simulink model "Integrate_SubMode_Motor"  (R2021b)
settings: Solver=FixedStepAuto  StartTime=0.0  StopTime=inf  FixedStep=0.01  RelTol=1e-3  EnableMultiTasking=on
values from neighbouring files (symbols this model uses):
  den_Gd = Gd.Den{:}    [para.m]
  Ki = 0.003    [para.m]
  Kp = 0.0001    [para.m]
  num_Gd = Gd.Num{:}    [para.m]
  rpm_scale = 1/12/4*60    (= 1.25)    [para.m]
  Wref = 4000    [para.m]
undefined symbols (not defined in the file or in its folder): dir, dist, pot2rpm
libraries: arduinolib x8, arduinosensorlib x5, simulink x4
settings Model: SimulationMode=external  ExtModeTrigDuration=2  Creator=user  LastModifiedBy=user
settings SolverCC: AutoInsertRateTranBlk=on
settings OptimizationCC: EnhancedBackFolding=on  PassReuseOutputArgsAs=Individual arguments  ZeroExternalMemoryAtStartup=off  ZeroInternalMemoryAtStartup=off  MaxStackSize=64  OptimizeBlockOrder=speed  DifferentSizesBufferReuse=on  OptimizationCustomize=off  EfficientTunableParamExpr=on
settings DebuggingCC: ParameterTunabilityLossMsg=error
settings HardwareCC: ProdBitPerInt=16  ProdBitPerPointer=16  ProdBitPerSizeT=16  ProdBitPerPtrDiffT=16  ProdLargestAtomicFloat=None  ProdWordSize=8  ProdHWDeviceType=Atmel->AVR
settings SFSimCC: MATLABDynamicMemAlloc=off
settings RTWCC: Description=Embedded Coder  SystemTargetFile=ert.tlc  HardwareBoard=Arduino Mega 2560  TemplateMakefile=ert_default_tmf  Toolchain=Arduino AVR  BuildConfiguration=Faster Runs
settings CodeAppCC: ForceParamTrailComments=on  IgnoreCustomStorageClasses=off  OperatorAnnotations=on  SimulinkDataObjDesc=on  SFDataObjDesc=on  InsertBlockDesc=on
settings ERTTargetCC: SupportContinuousTime=on  SupportVariableSizeSignals=on  ExtMode=on  ExtModeTransport=3  ExtModeStaticAlloc=on  ExtModeStaticAllocSize=2048  ExtModeMexFile=ext_xcp  ExtModeMexArgs=0 5 921600  ExtModeIntrfLevel=Level2 - Open

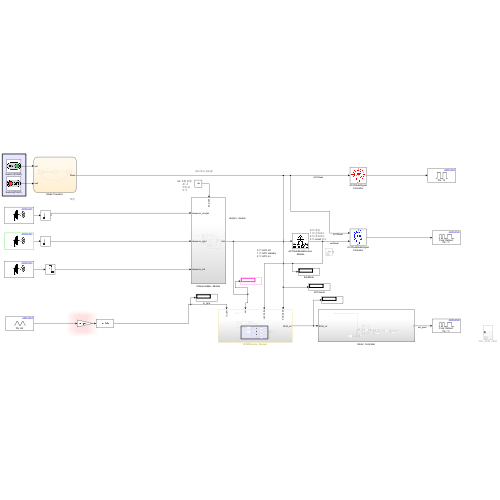
[thumbnail: Simulink's stored preview of the top-level diagram]
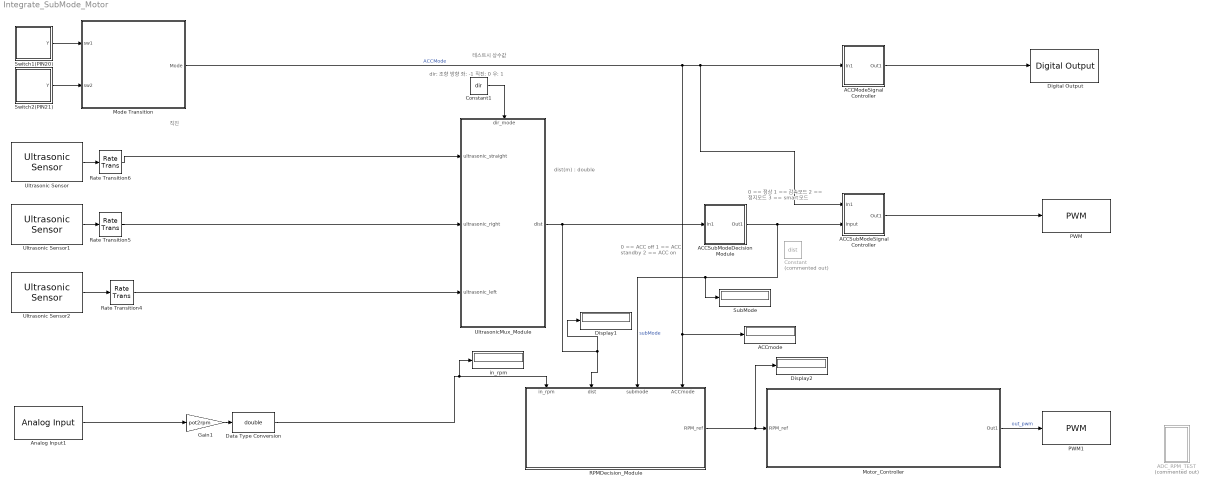
== system Integrate_SubMode_Motor ==
  note: dist(m) : double
  note: 테스트시 상수값
  note: 직진
  note: dir: 조향 방향
      |  	좌: -1
      |  	직진: 0
      |  	우: 1
  note: 0 == 정상
      | 1 == 감속모드
      | 2 == 정지모드
      | 3 == smart 모드
  note: 0 == ACC off
      | 1 == ACC standby
      | 2 == ACC on
  ACCModeSignal Controller : Subsystem
      mask Display: image('$imagefile'); % 변경하려면 툴스트립에 있는 "이미지 편집"을 사용하십시오.
  ACCSubModeDecision Module : Subsystem
      mask Display: image('$imagefile'); % 변경하려면 툴스트립에 있는 "이미지 편집"을 사용하십시오.
  ACCSubModeSignal Controller : Subsystem
      mask Display: image('$imagefile'); % 변경하려면 툴스트립에 있는 "이미지 편집"을 사용하십시오.
  ACCmode : Display
  ADC_RPM_TEST : Subsystem  Commented=on
  Analog Input1 : arduinolib/Analog Input  pinNumber=0  ReadResultsOnly=off  ConversionTriggerSource=Software  ExternalTriggerType=uint32( 0 )  OutputDataType=uint16  EnableConversionCompleteNotify=off  EnableOuputStatus=off  SampleTime=-1  blockPlatform=arduino
  Constant : Constant  Commented=on  Value=dist
  Constant1 : Constant  Value=dir
  Data Type Conversion : DataTypeConversion  OutDataTypeStr=double
  Digital Output : arduinolib/Digital Output  pinNumber=12  Direction=output  blockPlatform=arduino
  Display1 : Display
  Display2 : Display
  Gain1 : Gain  Gain=pot2rpm
  Mode Transition : Stateflow chart  TreatAsAtomicUnit=on
  Motor_Controller : Subsystem
  PWM : arduinolib/PWM  pinNumber=11  frequencyType=Default  desiredFrequency=490.2  achievableFrequency=490.2
  PWM1 : arduinolib/PWM  pinNumber=11  frequencyType=Default  desiredFrequency=490.2  achievableFrequency=490.2
  RPMDecision_Module : Subsystem
      settings: PortSchema="{\"entries\":[{\"content\":{\"sides\":[{\"content\":{\"connectorIds\":[]},\"type\":\"ConnectorPlacement.EquallySpacedRectSide\",\"uuid\":\"6ec364ce-34b2-4beb-b97a-f32003c79d6e\"},{\"content\":{\"connectorIds\":[\"Out1\"],\"side\":\"RIGHT\"},\"type\":\"ConnectorPlacement.EquallySpacedRectSide\",\"uuid\":\"dc876503-cb4c-4ae1-9014-14ad87bdb333\"},{\"content\":{\"connectorIds\":[\"In1\",\"In2\",\"In3\",\"In4\"],\"side\":\"TOP\"},\"type\":\"ConnectorPlacement.EquallySpacedRectSide\",\"uuid\":\"5447802f-a25d-4c34-9dc6-d7b36056ed0d\"}]},\"type\":\"ConnectorPlacement.EquallySpacedConnector\",\"uuid\":\"292fcb4a-6f45-4a66-adbd-fd22b6096994\"}],\"packageUris\":[\"http://schema.mathworks.com/mf0/Connector/R2020b\"],\"version\":\"1.0\"}"
  Rate Transition4 : RateTransition  Deterministic=off  OutPortSampleTime=0.03
  Rate Transition5 : RateTransition  Deterministic=off  OutPortSampleTime=0.03
  Rate Transition6 : RateTransition  Deterministic=off  OutPortSampleTime=0.03
  SubMode : Display
  Switch1(PIN20) : Subsystem
      mask Display: image('$imagefile'); % 변경하려면 툴스트립에 있는 "이미지 편집"을 사용하십시오.
  Switch2(PIN21) : Subsystem
      mask Display: image('$imagefile'); % 변경하려면 툴스트립에 있는 "이미지 편집"을 사용하십시오.
  Ultrasonic Sensor : arduinosensorlib/Ultrasonic Sensor  NumSignalPins=2  TrigPin=50  EchoPin=51  SignalPin=3  SampleTime_=0.1  blockPlatform=ARDUINO
      settings: SourceProductBaseCode=ARDUINO
  Ultrasonic Sensor1 : arduinosensorlib/Ultrasonic Sensor  NumSignalPins=2  TrigPin=48  EchoPin=49  SignalPin=3  SampleTime_=0.1  blockPlatform=ARDUINO
      settings: SourceProductBaseCode=ARDUINO
  Ultrasonic Sensor2 : arduinosensorlib/Ultrasonic Sensor  NumSignalPins=2  TrigPin=46  EchoPin=47  SignalPin=3  SampleTime_=0.1  blockPlatform=ARDUINO
      settings: SourceProductBaseCode=ARDUINO
  UltrasonicMux_Module : Subsystem
      settings: PortSchema="{\"entries\":[{\"content\":{\"sides\":[{\"content\":{\"connectorIds\":[\"In1\",\"In2\",\"In3\"]},\"type\":\"ConnectorPlacement.EquallySpacedRectSide\",\"uuid\":\"5f4ad8f0-04c3-4479-9dfd-33641402f242\"},{\"content\":{\"connectorIds\":[\"Out1\"],\"side\":\"RIGHT\"},\"type\":\"ConnectorPlacement.EquallySpacedRectSide\",\"uuid\":\"c4451af6-64c8-402e-8ffe-feeed5b209e6\"},{\"content\":{\"connectorIds\":[\"In4\"],\"side\":\"TOP\"},\"type\":\"ConnectorPlacement.EquallySpacedRectSide\",\"uuid\":\"4be8f8c7-8102-4379-8072-e8a8027f489d\"}]},\"type\":\"ConnectorPlacement.EquallySpacedConnector\",\"uuid\":\"2bd08bb9-e7f4-4004-b808-4b0f9daf5a96\"}],\"packageUris\":[\"http://schema.mathworks.com/mf0/Connector/R2020b\"],\"version\":\"1.0\"}"
  in_rpm : Display
  wires:
  Gain1/1 -> Data Type Conversion/1
  Data Type Conversion/1 -> in_rpm/1, RPMDecision_Module/1(in_rpm)
  Constant1/1 -> UltrasonicMux_Module/4(dir_mode)
  Ultrasonic Sensor2/1 -> Rate Transition4/1
  Ultrasonic Sensor1/1 -> Rate Transition5/1
  Ultrasonic Sensor/1 -> Rate Transition6/1
  Rate Transition6/1 -> UltrasonicMux_Module/1(ultrasonic_straight)
  Rate Transition5/1 -> UltrasonicMux_Module/2(ultrasonic_right)
  Rate Transition4/1 -> UltrasonicMux_Module/3(ultrasonic_left)
  Analog Input1/1 -> Gain1/1
  Motor_Controller/1(Out1) -> PWM1/1  "out_pwm"
  RPMDecision_Module/1(RPM_ref) -> Display2/1, Motor_Controller/1(RPM_ref)
  UltrasonicMux_Module/1(dist) -> ACCSubModeDecision Module/1(In1), RPMDecision_Module/2(dist), Display1/1
  Switch2(PIN21)/1(Y) -> Mode Transition/2(sw2)
  Switch1(PIN20)/1(Y) -> Mode Transition/1(sw1)
  Mode Transition/1(Mode) -> ACCSubModeSignal Controller/1(In1), ACCModeSignal Controller/1(In1), ACCmode/1, RPMDecision_Module/4(ACCmode)  "ACCMode"
  ACCSubModeDecision Module/1(Out1) -> ACCSubModeSignal Controller/2(Input), RPMDecision_Module/3(submode), SubMode/1  "subMode"
  ACCModeSignal Controller/1(Out1) -> Digital Output/1
  ACCSubModeSignal Controller/1(Out1) -> PWM/1

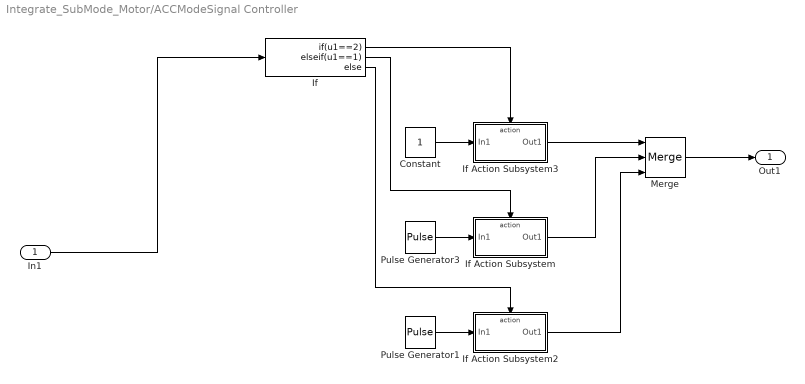
== system Integrate_SubMode_Motor/ACCModeSignal Controller ==
  In1 : Inport
  Constant : Constant
  If : If  IfExpression=u1==2  ElseIfExpressions=u1==1
  If Action Subsystem : Subsystem  TreatAsAtomicUnit=on
  If Action Subsystem2 : Subsystem  TreatAsAtomicUnit=on
  If Action Subsystem3 : Subsystem  TreatAsAtomicUnit=on
  Merge : Merge  Inputs=3
  Pulse Generator1 : DiscretePulseGenerator  PulseType=Time based  Period=1  PulseWidth=50  SampleTime=-1
  Pulse Generator3 : DiscretePulseGenerator  PulseType=Time based  Period=0.2  PulseWidth=50  SampleTime=-1
  Out1 : Outport
  wires:
  If Action Subsystem2/1(Out1) -> Merge/3
  Pulse Generator1/1 -> If Action Subsystem2/1(In1)
  Pulse Generator3/1 -> If Action Subsystem/1(In1)
  Merge/1 -> Out1/1
  If Action Subsystem/1(Out1) -> Merge/2
  If/1 -> If Action Subsystem3/Action
  If/2 -> If Action Subsystem/Action
  Constant/1 -> If Action Subsystem3/1(In1)
  If/3 -> If Action Subsystem2/Action
  If Action Subsystem3/1(Out1) -> Merge/1
  In1/1 -> If/1

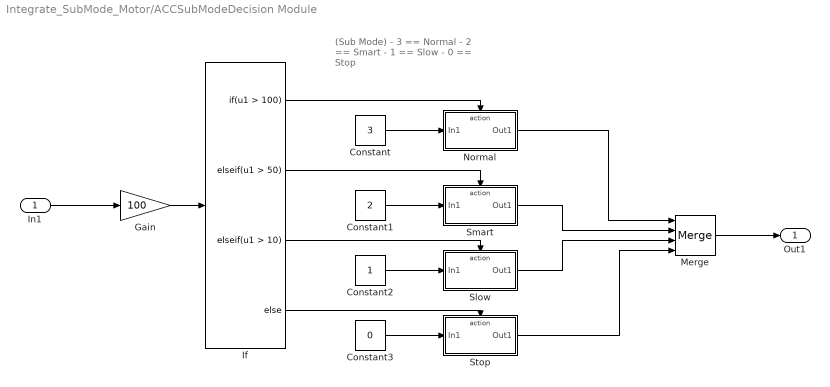
== system Integrate_SubMode_Motor/ACCSubModeDecision Module ==
  note: (Sub Mode)
      | - 3 == Normal
      | - 2 == Smart
      | - 1 == Slow
      | - 0 == Stop
  In1 : Inport
  Constant : Constant  Value=3
  Constant1 : Constant  Value=2
  Constant2 : Constant
  Constant3 : Constant  Value=0
  Gain : Gain  Gain=100
  If : If  IfExpression=u1 > 100  ElseIfExpressions=u1 > 50, u1 > 10
  Merge : Merge  Inputs=4
  "Normal " : Subsystem  TreatAsAtomicUnit=on
  Slow : Subsystem  TreatAsAtomicUnit=on
  Smart : Subsystem  TreatAsAtomicUnit=on
  Stop : Subsystem  TreatAsAtomicUnit=on
  Out1 : Outport
  wires:
  Slow/1(Out1) -> Merge/3
  Smart/1(Out1) -> Merge/2
  "Normal "/1(Out1) -> Merge/1
  Gain/1 -> If/1
  Constant2/1 -> Slow/1(In1)
  Constant/1 -> "Normal "/1(In1)
  In1/1 -> Gain/1
  Merge/1 -> Out1/1
  If/1 -> "Normal "/Action
  Constant3/1 -> Stop/1(In1)
  If/2 -> Smart/Action
  If/3 -> Slow/Action
  If/4 -> Stop/Action
  Stop/1(Out1) -> Merge/4
  Constant1/1 -> Smart/1(In1)

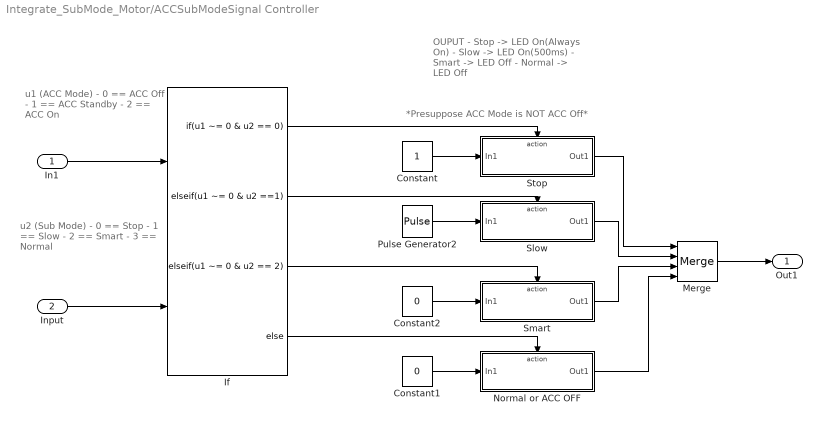
== system Integrate_SubMode_Motor/ACCSubModeSignal Controller ==
  note: u2 (Sub Mode)
      | - 0 == Stop
      | - 1 == Slow
      | - 2 == Smart
      | - 3 == Normal
  note: u1 (ACC Mode)
      | - 0 == ACC Off
      | - 1 == ACC Standby
      | - 2 ==  ACC On
  note: OUPUT
      | - Stop -> LED On(Always On)
      | - Slow -> LED On(500ms)
      | - Smart -> LED Off
      | - Normal -> LED Off
  note: *Presuppose ACC Mode is NOT ACC Off*
  In1 : Inport
  Input : Inport  Port=2
  Constant : Constant
  Constant1 : Constant  Value=0
  Constant2 : Constant  Value=0
  If : If  NumInputs=2  IfExpression=u1 ~= 0 & u2 == 0  ElseIfExpressions=u1 ~= 0 & u2 ==1, u1 ~= 0 & u2 == 2
  Merge : Merge  Inputs=4
  Normal or ACC OFF : Subsystem  TreatAsAtomicUnit=on
  Pulse Generator2 : DiscretePulseGenerator  PulseType=Time based  Period=0.2  PulseWidth=50  SampleTime=-1
  Slow : Subsystem  TreatAsAtomicUnit=on
  Smart : Subsystem  TreatAsAtomicUnit=on
  Stop : Subsystem  TreatAsAtomicUnit=on
  Out1 : Outport
  wires:
  Constant1/1 -> Normal or ACC OFF/1(In1)
  Pulse Generator2/1 -> Slow/1(In1)
  Merge/1 -> Out1/1
  Slow/1(Out1) -> Merge/2
  Constant/1 -> Stop/1(In1)
  Stop/1(Out1) -> Merge/1
  In1/1 -> If/1
  Input/1 -> If/2
  Constant2/1 -> Smart/1(In1)
  Normal or ACC OFF/1(Out1) -> Merge/4
  Smart/1(Out1) -> Merge/3
  If/1 -> Stop/Action
  If/2 -> Slow/Action
  If/3 -> Smart/Action
  If/4 -> Normal or ACC OFF/Action

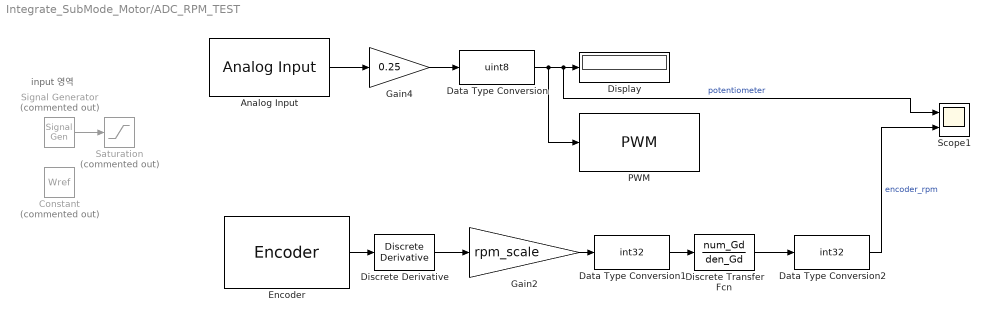
== system Integrate_SubMode_Motor/ADC_RPM_TEST ==
  note: input 영역
  Analog Input : arduinolib/Analog Input  pinNumber=0  ReadResultsOnly=off  ConversionTriggerSource=Software  ExternalTriggerType=uint32( 0 )  OutputDataType=uint16  EnableConversionCompleteNotify=off  EnableOuputStatus=off  SampleTime=-1  blockPlatform=arduino
  Constant : Constant  Commented=on  Value=Wref
  Data Type Conversion : DataTypeConversion  OutDataTypeStr=uint8
  Data Type Conversion1 : DataTypeConversion  OutDataTypeStr=int32
  Data Type Conversion2 : DataTypeConversion  OutDataTypeStr=int32
  Discrete Transfer Fcn : DiscreteTransferFcn  Numerator=num_Gd  Denominator=den_Gd
  Discrete Derivative : simulink/Discrete/Discrete Derivative  gainval=1.0  ICPrevScaledInput=0.0  OutMin=[]  OutMax=[]  OutDataType=fixdt(1, 16)  OutScaling=2^-10  DoSatur=off
  Display : Display
  Encoder : arduinosensorlib/Encoder  InputA=18  InputB=19  Mode=No reset  SampleTime=-1
      settings: SourceProductBaseCode=ARDUINO
  Gain2 : Gain  Gain=rpm_scale  OutDataTypeStr=double
  Gain4 : Gain  Gain=0.25
  PWM : arduinolib/PWM  pinNumber=11  frequencyType=Default  desiredFrequency=490.2  achievableFrequency=490.2
  Saturation : Saturate  Commented=on  UpperLimit=inf  LowerLimit=0
  Scope1 : Scope  NumInputPorts=2
  Signal Generator : SignalGenerator  Commented=on  Amplitude=5300  Frequency=0.1  Units=rad/sec
  wires:
  Discrete Transfer Fcn/1 -> Data Type Conversion2/1
  Encoder/1 -> Discrete Derivative/1
  Analog Input/1 -> Gain4/1
  Data Type Conversion1/1 -> Discrete Transfer Fcn/1
  Gain4/1 -> Data Type Conversion/1
  Data Type Conversion/1 -> PWM/1, Scope1/1, Display/1  "potentiometer"
  Discrete Derivative/1 -> Gain2/1
  Gain2/1 -> Data Type Conversion1/1
  Data Type Conversion2/1 -> Scope1/2  "encoder_rpm"
  Signal Generator/1 -> Saturation/1

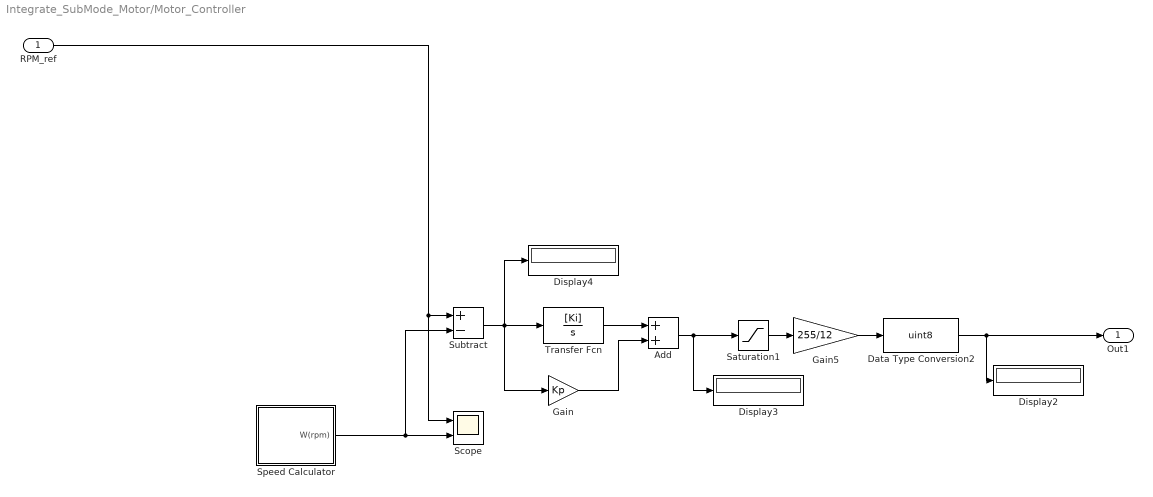
== system Integrate_SubMode_Motor/Motor_Controller ==
  RPM_ref : Inport
  Add : Sum
  Data Type Conversion2 : DataTypeConversion  OutDataTypeStr=uint8
  Display2 : Display
  Display3 : Display
  Display4 : Display
  Gain : Gain  Gain=Kp
  Gain5 : Gain  Gain=255/12
  Saturation1 : Saturate  UpperLimit=12  LowerLimit=0
  Scope : Scope  NumInputPorts=2
  Speed Calculator : Subsystem
  Subtract : Sum  Inputs=+-
  Transfer Fcn : TransferFcn  Numerator=[Ki]  Denominator=[1 0]
  Out1 : Outport
  wires:
  Data Type Conversion2/1 -> Out1/1, Display2/1
  Subtract/1 -> Display4/1, Transfer Fcn/1, Gain/1
  Speed Calculator/1(W(rpm)) -> Subtract/2, Scope/2
  Add/1 -> Display3/1, Saturation1/1
  Gain5/1 -> Data Type Conversion2/1
  Gain/1 -> Add/2
  Saturation1/1 -> Gain5/1
  Transfer Fcn/1 -> Add/1
  RPM_ref/1 -> Scope/1, Subtract/1

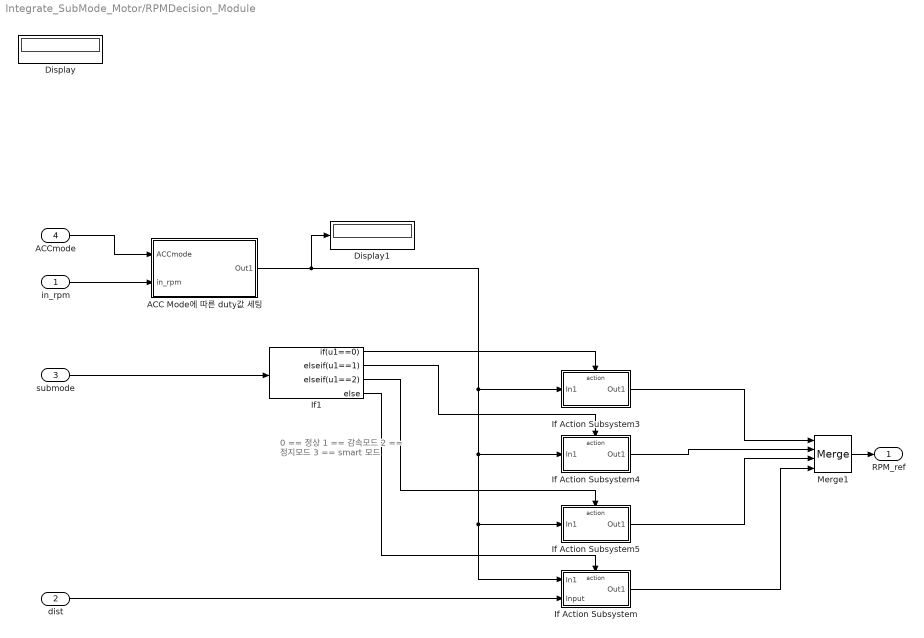
== system Integrate_SubMode_Motor/RPMDecision_Module ==
  note: 0 == 정상
      | 1 == 감속모드
      | 2 == 정지모드
      | 3 == smart 모드
  in_rpm : Inport
  dist : Inport  Port=2
  submode : Inport  Port=3
  ACCmode : Inport  Port=4
  ACC Mode에 따른 duty값 세팅 : Subsystem
  Display : Display
  Display1 : Display
  If Action Subsystem : Subsystem  TreatAsAtomicUnit=on
  If Action Subsystem3 : Subsystem  TreatAsAtomicUnit=on
  If Action Subsystem4 : Subsystem  TreatAsAtomicUnit=on
  If Action Subsystem5 : Subsystem  TreatAsAtomicUnit=on
  If1 : If  IfExpression=u1==0  ElseIfExpressions=u1==1, u1==2
  Merge1 : Merge  Inputs=4
  RPM_ref : Outport
  wires:
  in_rpm/1 -> ACC Mode에 따른 duty값 세팅/2(in_rpm)
  If Action Subsystem5/1(Out1) -> Merge1/3
  submode/1 -> If1/1
  If Action Subsystem4/1(Out1) -> Merge1/2
  If1/2 -> If Action Subsystem4/Action
  dist/1 -> If Action Subsystem/2(Input)
  If Action Subsystem3/1(Out1) -> Merge1/1
  If1/3 -> If Action Subsystem5/Action
  If1/1 -> If Action Subsystem3/Action
  ACC Mode에 따른 duty값 세팅/1(Out1) -> Display1/1, If Action Subsystem/1(In1), If Action Subsystem5/1(In1), If Action Subsystem4/1(In1), If Action Subsystem3/1(In1)
  If1/4 -> If Action Subsystem/Action
  ACCmode/1 -> ACC Mode에 따른 duty값 세팅/1(ACCmode)
  Merge1/1 -> RPM_ref/1
  If Action Subsystem/1(Out1) -> Merge1/4

== system Integrate_SubMode_Motor/Switch1(PIN20) ==
  Detect Increase : simulink/Logic and Bit Operations/Detect Increase  vinit=0.0  OutDataTypeStr=boolean
  Display2 : Display
  External Interrupt : arduinolib/External Interrupt  Pin=20  PullUp=on  Mode=FALLING  InterruptSimulationInput=off
      settings: SourceProductBaseCode=ARDUINO
  Function-Call Subsystem : Subsystem  TreatAsAtomicUnit=on
  Rate Transition : RateTransition  Integrity=off  Deterministic=off
  Y : Outport
  wires:
  Function-Call Subsystem/1(y) -> Rate Transition/1
  Rate Transition/1 -> Display2/1, Detect Increase/1
  External Interrupt/1 -> Function-Call Subsystem/Trigger
  Detect Increase/1 -> Y/1

== system Integrate_SubMode_Motor/Switch2(PIN21) ==
  Detect Increase1 : simulink/Logic and Bit Operations/Detect Increase  vinit=0.0  OutDataTypeStr=uint8
  Display3 : Display
  External Interrupt1 : arduinolib/External Interrupt  Pin=21  PullUp=on  Mode=FALLING  InterruptSimulationInput=off
      settings: SourceProductBaseCode=ARDUINO
  Function-Call Subsystem1 : Subsystem  TreatAsAtomicUnit=on
  Rate Transition1 : RateTransition  Deterministic=off
  Y : Outport
  wires:
  Function-Call Subsystem1/1(Out1) -> Rate Transition1/1
  Rate Transition1/1 -> Display3/1, Detect Increase1/1
  External Interrupt1/1 -> Function-Call Subsystem1/Trigger
  Detect Increase1/1 -> Y/1

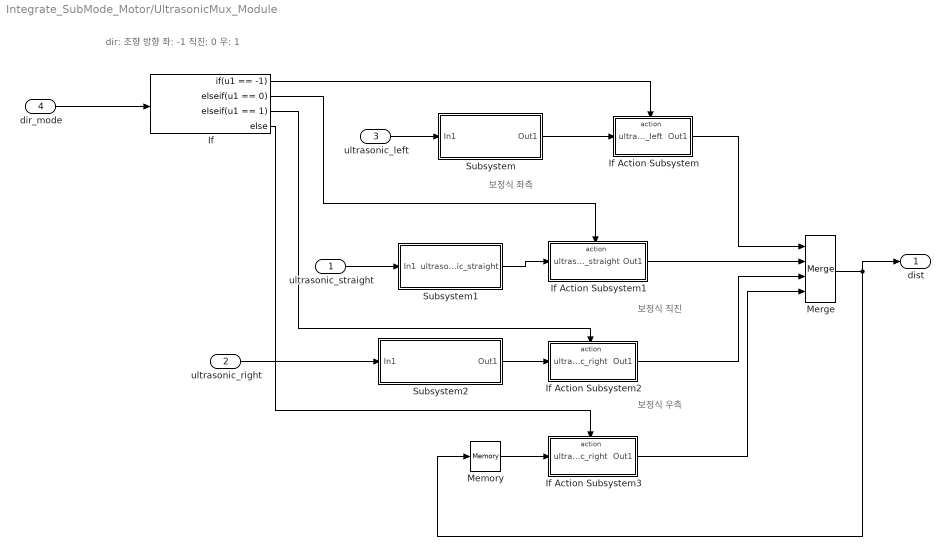
== system Integrate_SubMode_Motor/UltrasonicMux_Module ==
  note: 보정식 직진
  note: 보정식 좌측
  note: dir: 조향 방향
      |  	좌: -1
      |  	직진: 0
      |  	우: 1
  note: 보정식 우측
  ultrasonic_straight : Inport
  ultrasonic_right : Inport  Port=2
  ultrasonic_left : Inport  Port=3
  dir_mode : Inport  Port=4
  If : If  IfExpression=u1 == -1  ElseIfExpressions=u1 == 0, u1 == 1
  If Action Subsystem : Subsystem  TreatAsAtomicUnit=on
  If Action Subsystem1 : Subsystem  TreatAsAtomicUnit=on
  If Action Subsystem2 : Subsystem  TreatAsAtomicUnit=on
  If Action Subsystem3 : Subsystem  TreatAsAtomicUnit=on
  Memory : Memory
  Merge : Merge  Inputs=4
  Subsystem : Subsystem
  Subsystem1 : Subsystem
  Subsystem2 : Subsystem
  dist : Outport
  wires:
  dir_mode/1 -> If/1
  If/1 -> If Action Subsystem/Action
  ultrasonic_left/1 -> Subsystem/1(In1)
  If/2 -> If Action Subsystem1/Action
  ultrasonic_right/1 -> Subsystem2/1(In1)
  If Action Subsystem/1(Out1) -> Merge/1
  Merge/1 -> dist/1, Memory/1
  Subsystem/1(Out1) -> If Action Subsystem/1(ultrasonic_left)
  Subsystem1/1(ultrasonic_straight) -> If Action Subsystem1/1(ultrasonic_straight)
  ultrasonic_straight/1 -> Subsystem1/1(In1)
  If Action Subsystem1/1(Out1) -> Merge/2
  If Action Subsystem2/1(Out1) -> Merge/3
  Subsystem2/1(Out1) -> If Action Subsystem2/1(ultrasonic_right)
  If/3 -> If Action Subsystem2/Action
  Memory/1 -> If Action Subsystem3/1(ultrasonic_right)
  If/4 -> If Action Subsystem3/Action
  If Action Subsystem3/1(Out1) -> Merge/4

== system Integrate_SubMode_Motor/ACCModeSignal Controller/If Action Subsystem ==
  In1 : Inport
  Action Port : ActionPort
  Out1 : Outport
  wires:
  In1/1 -> Out1/1

== system Integrate_SubMode_Motor/ACCModeSignal Controller/If Action Subsystem2 ==
  In1 : Inport
  Action Port : ActionPort
  Out1 : Outport
  wires:
  In1/1 -> Out1/1

== system Integrate_SubMode_Motor/ACCModeSignal Controller/If Action Subsystem3 ==
  In1 : Inport
  Action Port : ActionPort
  Out1 : Outport
  wires:
  In1/1 -> Out1/1

== system Integrate_SubMode_Motor/ACCSubModeDecision Module/Normal  ==
  In1 : Inport
  Action Port : ActionPort
  Out1 : Outport
  wires:
  In1/1 -> Out1/1

== system Integrate_SubMode_Motor/ACCSubModeDecision Module/Slow ==
  In1 : Inport
  Action Port : ActionPort
  Out1 : Outport
  wires:
  In1/1 -> Out1/1

== system Integrate_SubMode_Motor/ACCSubModeDecision Module/Smart ==
  In1 : Inport
  Action Port : ActionPort
  Out1 : Outport
  wires:
  In1/1 -> Out1/1

== system Integrate_SubMode_Motor/ACCSubModeDecision Module/Stop ==
  In1 : Inport
  Action Port : ActionPort
  Out1 : Outport
  wires:
  In1/1 -> Out1/1

== system Integrate_SubMode_Motor/ACCSubModeSignal Controller/Normal or ACC OFF ==
  In1 : Inport
  Action Port : ActionPort
  Out1 : Outport
  wires:
  In1/1 -> Out1/1

== system Integrate_SubMode_Motor/ACCSubModeSignal Controller/Slow ==
  In1 : Inport
  Action Port : ActionPort
  Out1 : Outport
  wires:
  In1/1 -> Out1/1

== system Integrate_SubMode_Motor/ACCSubModeSignal Controller/Smart ==
  In1 : Inport
  Action Port : ActionPort
  Out1 : Outport
  wires:
  In1/1 -> Out1/1

== system Integrate_SubMode_Motor/ACCSubModeSignal Controller/Stop ==
  In1 : Inport
  Action Port : ActionPort
  Out1 : Outport
  wires:
  In1/1 -> Out1/1

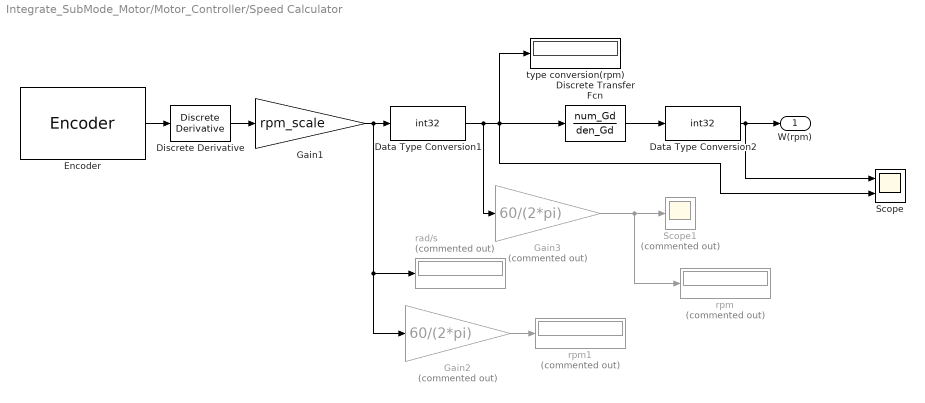
== system Integrate_SubMode_Motor/Motor_Controller/Speed Calculator ==
  Data Type Conversion1 : DataTypeConversion  OutDataTypeStr=int32
  Data Type Conversion2 : DataTypeConversion  OutDataTypeStr=int32
  Discrete Transfer Fcn : DiscreteTransferFcn  Numerator=num_Gd  Denominator=den_Gd
  Discrete Derivative : simulink/Discrete/Discrete Derivative  gainval=1.0  ICPrevScaledInput=0.0  OutMin=[]  OutMax=[]  OutDataType=fixdt(1, 16)  OutScaling=2^-10  DoSatur=off
  Encoder : arduinosensorlib/Encoder  InputA=18  InputB=19  Mode=No reset  SampleTime=-1
      settings: SourceProductBaseCode=ARDUINO
  Gain1 : Gain  Gain=rpm_scale  OutDataTypeStr=double
  Gain2 : Gain  Commented=on  Gain=60/(2*pi)  OutDataTypeStr=double
  Gain3 : Gain  Commented=on  Gain=60/(2*pi)  OutDataTypeStr=double
  Scope : Scope  NumInputPorts=2
  Scope1 : Scope  Commented=on
  rad/s : Display  Commented=on
  rpm : Display  Commented=on
  rpm1 : Display  Commented=on
  type conversion(rpm) : Display
  W(rpm) : Outport
  wires:
  Gain3/1 -> rpm/1, Scope1/1
  Gain2/1 -> rpm1/1
  Gain1/1 -> rad/s/1, Gain2/1, Data Type Conversion1/1
  Data Type Conversion1/1 -> type conversion(rpm)/1, Discrete Transfer Fcn/1, Scope/2, Gain3/1
  Discrete Derivative/1 -> Gain1/1
  Encoder/1 -> Discrete Derivative/1
  Discrete Transfer Fcn/1 -> Data Type Conversion2/1
  Data Type Conversion2/1 -> Scope/1, W(rpm)/1

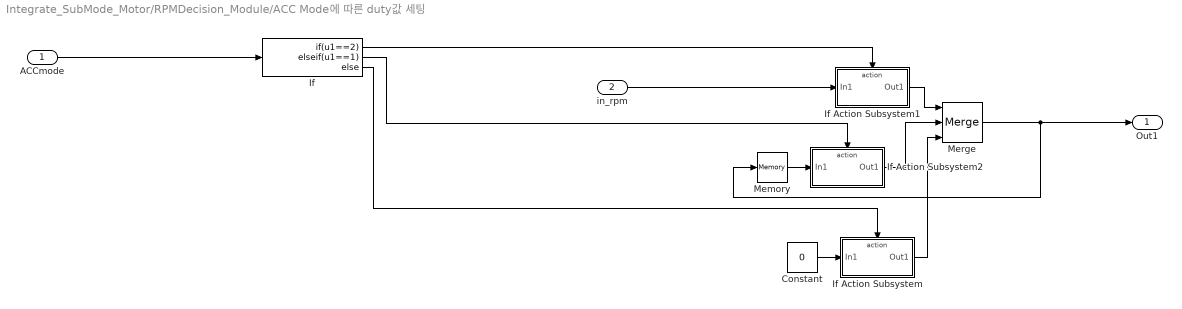
== system Integrate_SubMode_Motor/RPMDecision_Module/ACC Mode에 따른 duty값 세팅 ==
  ACCmode : Inport
  in_rpm : Inport  Port=2
  Constant : Constant  Value=0  OutDataTypeStr=double
  If : If  IfExpression=u1==2  ElseIfExpressions=u1==1
  If Action Subsystem : Subsystem  TreatAsAtomicUnit=on
  If Action Subsystem1 : Subsystem  TreatAsAtomicUnit=on
  If Action Subsystem2 : Subsystem  TreatAsAtomicUnit=on
  Memory : Memory
  Merge : Merge  Inputs=3
  Out1 : Outport
  wires:
  Constant/1 -> If Action Subsystem/1(In1)
  in_rpm/1 -> If Action Subsystem1/1(In1)
  If/2 -> If Action Subsystem2/Action
  If/3 -> If Action Subsystem/Action
  Memory/1 -> If Action Subsystem2/1(In1)
  Merge/1 -> Memory/1, Out1/1
  If/1 -> If Action Subsystem1/Action
  If Action Subsystem1/1(Out1) -> Merge/1
  If Action Subsystem2/1(Out1) -> Merge/2
  If Action Subsystem/1(Out1) -> Merge/3
  ACCmode/1 -> If/1

== system Integrate_SubMode_Motor/RPMDecision_Module/If Action Subsystem ==
  In1 : Inport
  Input : Inport  Port=2
  Action Port : ActionPort  ActionPortLabel=else
  Product : Product
  Out1 : Outport
  wires:
  In1/1 -> Product/1
  Input/1 -> Product/2
  Product/1 -> Out1/1

== system Integrate_SubMode_Motor/RPMDecision_Module/If Action Subsystem3 ==
  In1 : Inport
  Action Port : ActionPort  ActionPortLabel=if(u1==0)
  Out1 : Outport  OutDataTypeStr=double
  wires:
  In1/1 -> Out1/1

== system Integrate_SubMode_Motor/RPMDecision_Module/If Action Subsystem4 ==
  In1 : Inport
  Action Port : ActionPort  ActionPortLabel=elseif(u1==1)
  Gain : Gain  Gain=0.5  OutDataTypeStr=double
  Out1 : Outport  OutDataTypeStr=double
  wires:
  In1/1 -> Gain/1
  Gain/1 -> Out1/1

== system Integrate_SubMode_Motor/RPMDecision_Module/If Action Subsystem5 ==
  In1 : Inport
  Action Port : ActionPort  ActionPortLabel=elseif( u1==2)
  Gain : Gain  Gain=0  OutDataTypeStr=double
  Out1 : Outport
  wires:
  In1/1 -> Gain/1
  Gain/1 -> Out1/1

== system Integrate_SubMode_Motor/Switch1(PIN20)/Function-Call Subsystem ==
  function : TriggerPort  TriggerType=function-call  VariantControl=(inherit)
  Constant : Constant
  Sum : Sum  Inputs=|++
  Unit Delay : UnitDelay  SampleTime=-1  HasFrameUpgradeWarning=on
  y : Outport
  wires:
  Unit Delay/1 -> Sum/2
  Constant/1 -> Sum/1
  Sum/1 -> Unit Delay/1, y/1

== system Integrate_SubMode_Motor/Switch2(PIN21)/Function-Call Subsystem1 ==
  function : TriggerPort  TriggerType=function-call  VariantControl=(inherit)
  Constant : Constant
  Sum : Sum  Inputs=|++
  Unit Delay : UnitDelay  SampleTime=-1  HasFrameUpgradeWarning=on
  Out1 : Outport
  wires:
  Sum/1 -> Unit Delay/1, Out1/1
  Unit Delay/1 -> Sum/2
  Constant/1 -> Sum/1

== system Integrate_SubMode_Motor/UltrasonicMux_Module/If Action Subsystem ==
  ultrasonic_left : Inport
  Action Port : ActionPort  ActionPortLabel=if(u1 == -1)
  Out1 : Outport
  wires:
  ultrasonic_left/1 -> Out1/1

== system Integrate_SubMode_Motor/UltrasonicMux_Module/If Action Subsystem1 ==
  ultrasonic_straight : Inport
  Action Port : ActionPort  ActionPortLabel=elseif(u1 == 0)
  Out1 : Outport
  wires:
  ultrasonic_straight/1 -> Out1/1

== system Integrate_SubMode_Motor/UltrasonicMux_Module/If Action Subsystem2 ==
  ultrasonic_right : Inport
  Action Port : ActionPort  ActionPortLabel=elseif( u1 == 1)
  Out1 : Outport
  wires:
  ultrasonic_right/1 -> Out1/1

== system Integrate_SubMode_Motor/UltrasonicMux_Module/If Action Subsystem3 ==
  ultrasonic_right : Inport
  Action Port : ActionPort  ActionPortLabel=else
  Out1 : Outport
  wires:
  ultrasonic_right/1 -> Out1/1

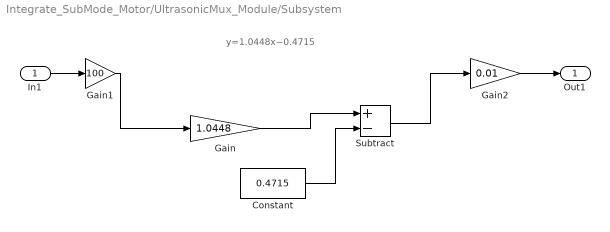
== system Integrate_SubMode_Motor/UltrasonicMux_Module/Subsystem ==
  note: y=1.0448x−0.4715
  In1 : Inport
  Constant : Constant  Value=0.4715
  Gain : Gain  Gain=1.0448
  Gain1 : Gain  Gain=100
  Gain2 : Gain  Gain=0.01
  Subtract : Sum  Inputs=+-
  Out1 : Outport
  wires:
  In1/1 -> Gain1/1
  Gain/1 -> Subtract/1
  Constant/1 -> Subtract/2
  Gain1/1 -> Gain/1
  Subtract/1 -> Gain2/1
  Gain2/1 -> Out1/1

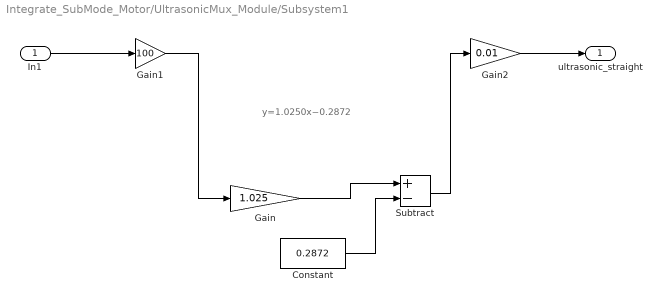
== system Integrate_SubMode_Motor/UltrasonicMux_Module/Subsystem1 ==
  note: y=1.0250x−0.2872
  In1 : Inport
  Constant : Constant  Value=0.2872
  Gain : Gain  Gain=1.025
  Gain1 : Gain  Gain=100
  Gain2 : Gain  Gain=0.01
  Subtract : Sum  Inputs=+-
  ultrasonic_straight : Outport
  wires:
  Gain/1 -> Subtract/1
  Constant/1 -> Subtract/2
  In1/1 -> Gain1/1
  Gain1/1 -> Gain/1
  Gain2/1 -> ultrasonic_straight/1
  Subtract/1 -> Gain2/1

== system Integrate_SubMode_Motor/UltrasonicMux_Module/Subsystem2 ==
  note: y=1.01365272x−0.77147476
  In1 : Inport
  Constant : Constant  Value=0.771474
  Gain : Gain  Gain=1.013652
  Gain1 : Gain  Gain=100
  Gain2 : Gain  Gain=0.01
  Subtract : Sum  Inputs=+-
  Out1 : Outport
  wires:
  Gain/1 -> Subtract/1
  Constant/1 -> Subtract/2
  In1/1 -> Gain1/1
  Subtract/1 -> Gain2/1
  Gain1/1 -> Gain/1
  Gain2/1 -> Out1/1

== system Integrate_SubMode_Motor/RPMDecision_Module/ACC Mode에 따른 duty값 세팅/If Action Subsystem ==
  In1 : Inport
  Action Port : ActionPort  ActionPortLabel=else
  Out1 : Outport
  wires:
  In1/1 -> Out1/1

== system Integrate_SubMode_Motor/RPMDecision_Module/ACC Mode에 따른 duty값 세팅/If Action Subsystem1 ==
  In1 : Inport
  Action Port : ActionPort  ActionPortLabel=if(u1==2)
  Out1 : Outport
  wires:
  In1/1 -> Out1/1

== system Integrate_SubMode_Motor/RPMDecision_Module/ACC Mode에 따른 duty값 세팅/If Action Subsystem2 ==
  In1 : Inport
  Action Port : ActionPort  ActionPortLabel=elseif(u1==1)
  Out1 : Outport
  wires:
  In1/1 -> Out1/1

== stateflow chart Integrate_SubMode_Motor/Mode Transition ==
  state ACC_off
    Mode=0;
  state ACC_standby
    Mode=1;
  state ACC_active
    Mode=2;
  (default) -> ACC_off
  ACC_standby -> ACC_active [order 2] : [sw1==1 ]
  ACC_off -> ACC_standby : [sw1==1 ]
  ACC_standby -> ACC_off [order 1] : [sw2==1]
  ACC_active -> ACC_off : [sw1 == 1 || sw2 ==1]
  data: Mode output; sw1 input; sw2 input
